simulink model "testSineWavein"  (R2021b)
settings: Solver=VariableStepAuto  StartTime=0.0  StopTime=10.0  RelTol=1e-3
values from neighbouring files (symbols this model uses):
  ad = exp(-Ts*pd_param.a)    [measureFrequencyResponse.m]    (also in measureFrequencyResponse_pd.m)
  pd_param = struct()    [designPD_lead_compensator.m]    (also in init.m = designPD_lead_compensator(lc_param); pd_parameters.mat = )
  Ts = 0.001    [init.m]    (also in measureFrequencyResponse.m; measureFrequencyResponse_pd.m; system_parameters.mat)
libraries: simulink x1
settings Model: Creator=ssapkota  LastModifiedBy=ssapkota

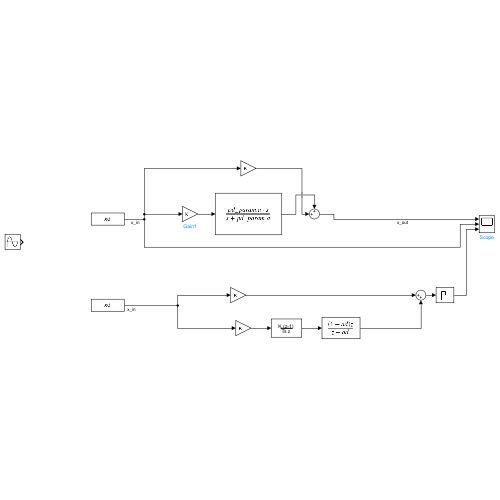
[thumbnail: Simulink's stored preview of the top-level diagram]
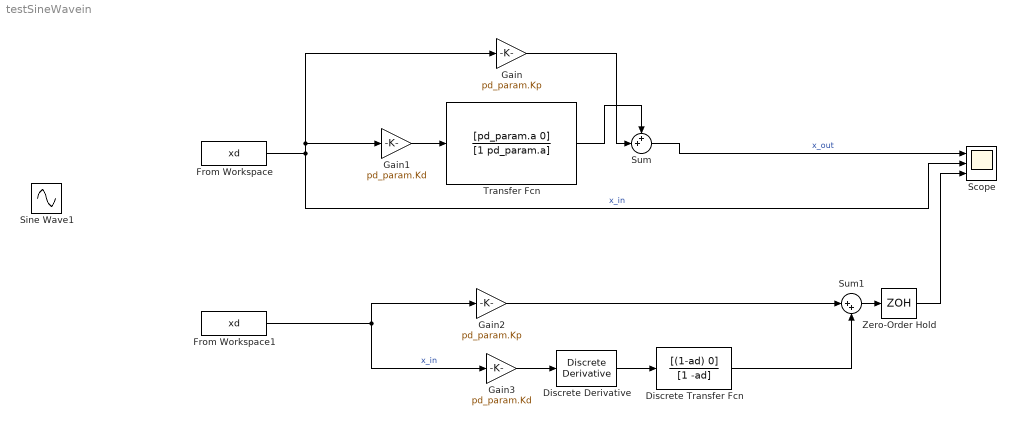
== system testSineWavein ==
  Discrete Transfer Fcn : DiscreteTransferFcn  Numerator=[(1-ad) 0]  Denominator=[1 -ad]  SampleTime=Ts
  Discrete Derivative : simulink/Discrete/Discrete Derivative  gainval=1.0  ICPrevScaledInput=0.0  OutMin=[]  OutMax=[]  OutDataType=fixdt(1, 16)  OutScaling=2^-10  DoSatur=off
  From Workspace : FromWorkspace  VariableName=xd
  From Workspace1 : FromWorkspace  VariableName=xd
  Gain : Gain  Gain=pd_param.Kp
  Gain1 : Gain  Gain=pd_param.Kd
  Gain2 : Gain  Gain=pd_param.Kp
  Gain3 : Gain  Gain=pd_param.Kd
  Scope : Scope  NumInputPorts=3
  Sine Wave1 : Sin  Frequency=50  SampleTime=0
  Sum : Sum  Inputs=++|
  Sum1 : Sum  Inputs=|++
  Transfer Fcn : TransferFcn  Numerator=[pd_param.a 0]  Denominator=[1 pd_param.a]
  Zero-Order Hold : ZeroOrderHold  SampleTime=-1
  wires:
  From Workspace/1 -> Gain1/1, Gain/1, Scope/2  "x_in"
  Gain1/1 -> Transfer Fcn/1
  Transfer Fcn/1 -> Sum/1
  Gain/1 -> Sum/2
  Sum/1 -> Scope/1  "x_out"
  Gain3/1 -> Discrete Derivative/1
  Discrete Derivative/1 -> Discrete Transfer Fcn/1
  From Workspace1/1 -> Gain3/1, Gain2/1  "x_in"
  Gain2/1 -> Sum1/1
  Discrete Transfer Fcn/1 -> Sum1/2
  Sum1/1 -> Zero-Order Hold/1
  Zero-Order Hold/1 -> Scope/3
